simulink model "mmc_model"  (R2023b)
settings: Solver=VariableStepAuto  StartTime=0.0  StopTime=simulation.tsim  RelTol=1e-3
values from neighbouring files (symbols this model uses):
  ab0_to_cell = inv(cell_to_2ab0)    [init_mmc.m]
  cell_to_2ab0 = kron(abc_to_ab0, abc_to_ab0)    [init_mmc.m]
  grid_to_cell = kron(eye(3), ones(3, 1))    [init_mmc.m]
  J = [0 -1; 1 0]    [init_mmc.m]
  machine_to_cell = kron(ones(3, 1), eye(3))    [init_mmc.m]
  volt_to_cell = [      [          1 0 0 0 0 0 ... (first row only)    [init_mmc.m]
undefined symbols (not defined in the file or in its folder): avi, clc, cpu, ctrl, currentControl, DiscIntNeverNeededParam, gfl, grid, load2, loadStep, machine, mmc, pq_ctrl, simulation, soa, stiffGrid, sync, testScenario
libraries: library x17, spsThreePhaseSeriesRLCBranchLib x16, eeGeneralControl x15, spsControlledVoltageSourceLib x15, simulink x11, spsThreePhaseVIMeasurementLib x10, spsGroundLib x9, eeDiscretePi x8, simulink_extras x8, spsabctodq0Lib x8, spsThreePhaseBreakerLib x7, spsdq0toabcLib x5
(part 1 of 3)
settings Model: SimulationMode=accelerator  Creator=ma1155716  LastModifiedBy=ma1155716

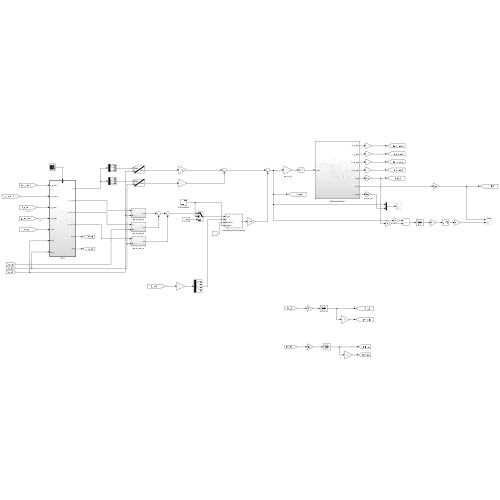
[thumbnail: Simulink's stored preview of the top-level diagram]
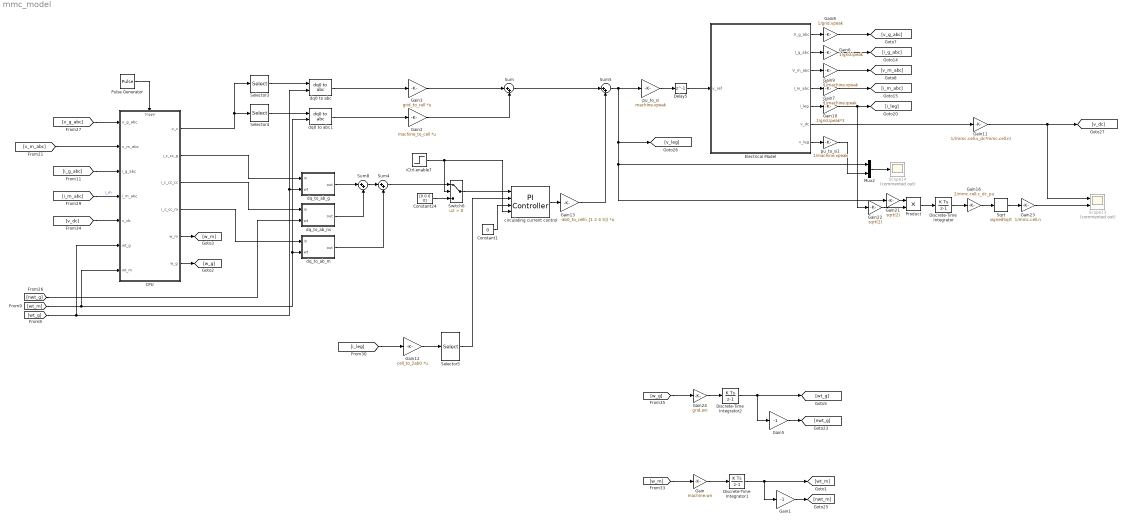
== system mmc_model ==
  CPU : Subsystem
  Constant1 : Constant  Value=0
  Constant24 : Constant  Value=[0 0 0 0]
  Delay5 : Delay  DelayLength=1  InitialCondition=0  SampleTime=simulation.ts
  Discrete-Time Integrator : DiscreteIntegrator  gainval=1  SampleTime=-1  ICPrevOutput=DiscIntNeverNeededParam  ICPrevScaledInput=DiscIntNeverNeededParam
  Discrete-Time Integrator1 : DiscreteIntegrator  gainval=1  SampleTime=-1  ICPrevOutput=DiscIntNeverNeededParam  ICPrevScaledInput=DiscIntNeverNeededParam
  Discrete-Time Integrator2 : DiscreteIntegrator  gainval=1  SampleTime=-1  ICPrevOutput=DiscIntNeverNeededParam  ICPrevScaledInput=DiscIntNeverNeededParam
  Electrical Model : Subsystem
  Gain : Gain  Gain=machine.wn
  Gain1 : Gain  Gain=-1
  Gain10 : Gain  Gain=1/grid.ipeak*3
  Gain11 : Gain  Gain=1/(mmc.cell.v_dc*mmc.cell.n)
  Gain12 : Gain  Gain=cell_to_2ab0  Multiplication=Matrix(K*u)
  Gain13 : Gain  Gain=-ab0_to_cell(:,[1 2 4 5])  Multiplication=Matrix(K*u)
  Gain16 : Gain  Gain=2/mmc.cell.c_dc_pu
  Gain2 : Gain  Gain=machine_to_cell  Multiplication=Matrix(K*u)
  Gain21 : Gain  Gain=sqrt(2)
  Gain22 : Gain  Gain=sqrt(2)
  Gain23 : Gain  Gain=1/mmc.cell.n
  Gain24 : Gain  Gain=grid.wn
  Gain3 : Gain  Gain=grid_to_cell  Multiplication=Matrix(K*u)
  Gain5 : Gain  Gain=-1
  Gain6 : Gain  Gain=1/grid.ipeak
  Gain7 : Gain  Gain=1/machine.ipeak
  Gain8 : Gain  Gain=1/grid.vpeak
  Gain9 : Gain  Gain=1/machine.vpeak
  Mux2 : Mux  Inputs=2
  Product : Product
  Pulse Generator : DiscretePulseGenerator  PulseType=Time based  Period=cpu.ts  PulseWidth=50
  Scope13 : Scope  Commented=on  NumInputPorts=2
  Scope14 : Scope  Commented=on
  Selector3 : Selector  InputPortWidth=5  IndexOptions=Index vector (dialog)  Indices=[1 2 5]  OutputSizes=1
  Selector4 : Selector  InputPortWidth=5  IndexOptions=Index vector (dialog)  Indices=[3 4 5]  OutputSizes=1
  Selector5 : Selector  InputPortWidth=9  IndexOptions=Index vector (dialog)  Indices=[1 2 4 5]  OutputSizes=1
  Sqrt : Sqrt  Operator=signedSqrt
  Sum{,4..5,8} (4 alike) : Sum  Inputs=|++
  Switch6 : Switch  Criteria=u2 > Threshold  SaturateOnIntegerOverflow=off  InputSameDT=off
  circulating current control : library/PI Controller  VariantControl=overcurr_ctrl.sel==1  kp=ctrl.grid.ictrl.kp  ti=1e6  Kaw=1
  dq0 to abc : spsdq0toabcLib/dq0 to abc  Alignment=Aligned with phase A axis
  dq0 to abc1 : spsdq0toabcLib/dq0 to abc  Alignment=Aligned with phase A axis
  dq_to_ab_g : Subsystem
  dq_to_ab_m : Subsystem
  dq_to_ab_ns : Subsystem
  iCtrl.enable7 : Step  Time=ctrl.grid.ictrl.enable
  pu_to_si : Gain  Gain=machine.vpeak
  pu_to_si1 : Gain  Gain=1/machine.vpeak
  wires:
  Electrical Model/2(I_g_abc) -> Gain6/1
  Electrical Model/4(I_m_abc) -> Gain7/1
  Pulse Generator/1 -> CPU/Trigger
  Discrete-Time Integrator2/1 -> [wt_g], Gain5/1
  Electrical Model/1(V_g_abc) -> Gain8/1
  Electrical Model/3(V_m_abc) -> Gain9/1
  dq0 to abc/1 -> Gain3/1
  dq0 to abc1/1 -> Gain2/1
  Selector3/1 -> dq0 to abc/1
  Selector4/1 -> dq0 to abc1/1
  CPU/1(v_c) -> Selector4/1, Selector3/1
  Gain3/1 -> Sum/1
  [i_g_abc] -> CPU/3(i_g_abc)
  pu_to_si/1 -> Delay5/1
  Electrical Model/5(i_leg) -> Gain10/1
  Gain6/1 -> [i_g_abc]
  Gain7/1 -> [i_m_abc]
  Gain8/1 -> [v_g_abc]
  Gain9/1 -> [v_m_abc]
  Gain10/1 -> Gain22/1, [i_leg]
  Gain5/1 -> [nwt_g]
  Discrete-Time Integrator1/1 -> [wt_m], Gain1/1
  Gain1/1 -> [nwt_m]
  Product/1 -> Discrete-Time Integrator/1
  [i_leg] -> Gain12/1
  Gain12/1 -> Selector5/1
  Discrete-Time Integrator/1 -> Gain16/1
  Gain16/1 -> Sqrt/1
  [v_dc] -> CPU/5(v_dc)
  Gain23/1 -> Scope13/2
  CPU/2(i_c_cc_g) -> dq_to_ab_g/1(in)
  [nwt_g] -> dq_to_ab_ns/2(wt)
  CPU/3(i_c_cc_cc) -> dq_to_ab_ns/1(in)
  CPU/4(i_c_cc_m) -> dq_to_ab_m/1(in)
  dq_to_ab_g/1(out) -> Sum8/1
  Sum8/1 -> Sum4/1
  dq_to_ab_ns/1(out) -> Sum8/2
  dq_to_ab_m/1(out) -> Sum4/2
  [wt_g] -> CPU/6(wt_g), dq0 to abc/2, dq_to_ab_g/2(wt)
  [wt_m] -> CPU/7(wt_m), dq_to_ab_m/2(wt), dq0 to abc1/2
  Constant1/1 -> circulating current control/3
  Sum4/1 -> Switch6/1
  Switch6/1 -> circulating current control/1
  iCtrl.enable7/1 -> Switch6/2, circulating current control/4
  Constant24/1 -> Switch6/3
  Sum/1 -> Sum5/1
  circulating current control/1 -> Gain13/1
  Gain11/1 -> [v_dc], Scope13/1
  Electrical Model/6(v_dc) -> Gain11/1
  Gain21/1 -> Product/1
  Gain22/1 -> Product/2
  Sqrt/1 -> Gain23/1
  Sum5/1 -> pu_to_si/1, [v_leg], Gain21/1, Mux2/1
  Electrical Model/7(v_leg) -> pu_to_si1/1
  pu_to_si1/1 -> Mux2/2
  Mux2/1 -> Scope14/1
  Gain2/1 -> Sum/2
  Selector5/1 -> circulating current control/2
  [i_m_abc] -> CPU/4(i_m_abc)  "i_m"
  CPU/5(w_m) -> [w_m]
  Gain/1 -> Discrete-Time Integrator1/1
  [w_m] -> Gain/1
  [v_g_abc] -> CPU/1(v_g_abc)
  Gain24/1 -> Discrete-Time Integrator2/1
  CPU/6(w_g) -> [w_g]
  [w_g] -> Gain24/1
  Gain13/1 -> Sum5/2
  Delay5/1 -> Electrical Model/1(v_ref)
  [v_m_abc] -> CPU/2(v_m_abc)

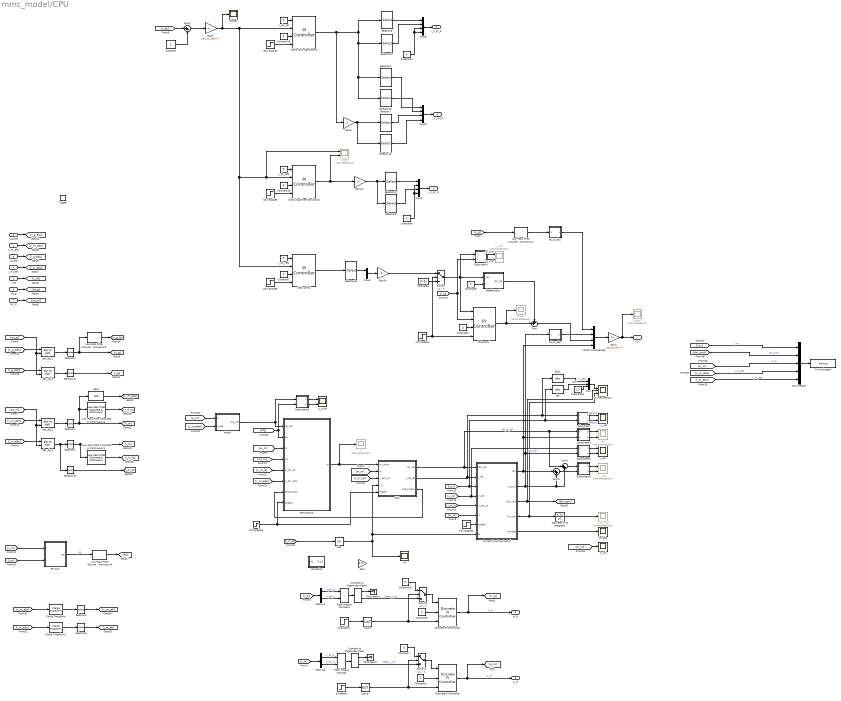
== system mmc_model/CPU ==
  v_g_abc : Inport
  v_m_abc : Inport  Port=2
  i_g_abc : Inport  Port=3
  i_m_abc : Inport  Port=4
  v_dc : Inport  Port=5
  wt_g : Inport  Port=6
  wt_m : Inport  Port=7
  Trigger : TriggerPort  VariantControl=(inherit)
  Abs : Abs  SaturateOnIntegerOverflow=off
  Bus Creator : BusCreator  Inputs=5
  Clarke Transform : eeTransforms/Clarke Transform  PowerInvariant=off
      settings: LibrarySourceBlock=|
      | ee_sl_lib/Mathematical
      | Transforms/Clarke Transform
  Clarke Transform1 : eeTransforms/Clarke Transform  PowerInvariant=off
      settings: LibrarySourceBlock=|
      | ee_sl_lib/Mathematical
      | Transforms/Clarke Transform
  Complex to Magnitude-Angle : ComplexToMagnitudeAngle
  Complex to Magnitude-Angle1 : ComplexToMagnitudeAngle
  Constant : Constant
  Constant{1..4,7..10,18..19} (10 alike) : Constant  Value=0
  Constant12 : Constant  Value=1.3
  Constant5 : Constant
  Constant6 : Constant  Value=[0 0]
  Current Limiting Control : Subsystem  Variant=on
  Demux1 : Demux  Outputs=2
  Demux6 : Demux  Outputs=2
  Discrete PI Controller : eeDiscretePi/Discrete PI Controller  Kp=ctrl.machine.pll.kp  Ki=ctrl.machine.pll.ti  Kaw=1  x0=ctrl.machine.pll.w0  Ts=-1
      settings: LibrarySourceBlock=ee_sl_lib/General Control/Discrete PI Controller
  Discrete PI Controller1 : eeDiscretePi/Discrete PI Controller  Kp=ctrl.grid.pll.kp  Ki=ctrl.grid.pll.ti  Kaw=1  x0=ctrl.grid.pll.w0  Ts=-1
      settings: LibrarySourceBlock=ee_sl_lib/General Control/Discrete PI Controller
  Discrete-Time Integrator : DiscreteIntegrator  gainval=1  SampleTime=-1  ICPrevOutput=DiscIntNeverNeededParam  ICPrevScaledInput=DiscIntNeverNeededParam
  GFM Control : Subsystem  Variant=on
  Gain : Gain  Gain=1.5
  Gain1 : Gain  Gain=volt_to_cell  Multiplication=Matrix(K*u)
  Gain12 : Gain  Gain=-1
  Gain14 : Gain  Gain=-1
  Gain5 : Gain  Gain=cell_to_2ab0  Multiplication=Matrix(K*u)
  Gain6 : Gain  Gain=-1
  Low-Pass Filter (Discrete or Continuous){1..4} (4 alike) : eeGeneralControl/Low-Pass Filter (Discrete or Continuous)  K=1  T=0.01  B=inf  A=-inf  init_option=Inherited from block input  x0=0  Ts=-1
  Low-Pass Filter (Discrete or Continuous)6 : eeGeneralControl/Low-Pass Filter (Discrete or Continuous)  K=1  T=0.1  B=inf  A=-inf  init_option=Inherited from block input  x0=0  Ts=-1
  Mux : Mux  Inputs=3
  Mux10 : Mux
  Mux6 : Mux  Inputs=2
  Mux8 : Mux
  Mux9 : Mux
  NOT1 : Logic  Operator=NOT  IconShape=distinctive  AllPortsSameDT=off  OutDataTypeStr=boolean
  NOT2 : Logic  Operator=NOT  IconShape=distinctive  AllPortsSameDT=off  OutDataTypeStr=boolean
  PQ Calc : Subsystem
  Real-Imag to Complex : RealImagToComplex
  Real-Imag to Complex1 : RealImagToComplex
  SOA : Subsystem
  Scope1 : Scope
  Scope5 : Scope  Commented=on
  Scope7 : Scope  Commented=on
  Scope8 : Scope  Commented=on  NumInputPorts=2
  Selector{1..5,17} (6 alike) : Selector  InputPortWidth=3  IndexOptions=Index vector (dialog)  Indices=[1 2]  OutputSizes=1
  Selector10 : Selector  InputPortWidth=9  IndexOptions=Index vector (dialog)  Indices=[8]  OutputSizes=1
  Selector11 : Selector  InputPortWidth=3  IndexOptions=Index vector (dialog)  Indices=[3]  OutputSizes=1
  Selector12 : Selector  InputPortWidth=9  IndexOptions=Index vector (dialog)  Indices=[3]  OutputSizes=1
  Selector13 : Selector  InputPortWidth=9  IndexOptions=Index vector (dialog)  Indices=[2]  OutputSizes=1
  Selector14 : Selector  InputPortWidth=9  IndexOptions=Index vector (dialog)  Indices=[5]  OutputSizes=1
  Selector15 : Selector  InputPortWidth=9  IndexOptions=Index vector (dialog)  Indices=[9]  OutputSizes=1
  Selector6 : Selector  InputPortWidth=9  IndexOptions=Index vector (dialog)  Indices=[1]  OutputSizes=1
  Selector7 : Selector  InputPortWidth=9  IndexOptions=Index vector (dialog)  Indices=[4]  OutputSizes=1
  Selector8 : Selector  InputPortWidth=9  IndexOptions=Index vector (dialog)  Indices=[7]  OutputSizes=1
  Selector9 : Selector  InputPortWidth=9  IndexOptions=Index vector (dialog)  Indices=[6]  OutputSizes=1
  Subsystem : Subsystem
  Subsystem1 : Subsystem
  Subsystem2 : Subsystem
  Subsystem3 : Subsystem
  Subsystem5 : Subsystem
  Subsystem6 : Subsystem
  Sum : Sum  Inputs=++|
  Sum1 : Sum  Inputs=|+-
  Sum3 : Sum  Inputs=|++
  Sum4 : Sum  Inputs=|++
  Switch : Switch  Criteria=u2 > Threshold  SaturateOnIntegerOverflow=off  InputSameDT=off
  Switch1 : Switch  Criteria=u2 > Threshold  SaturateOnIntegerOverflow=off  InputSameDT=off
  Switch2 : Switch  Criteria=u2 > Threshold  SaturateOnIntegerOverflow=off  InputSameDT=off
  Terminator1 : Terminator
  Terminator7 : Terminator
  To Workspace : ToWorkspace  VariableName=simout  SaveFormat=Timeseries  SampleTime=-1
  Vector Concatenate : Concatenate  NumInputs=4
  ab_to_ab0 : Subsystem
  ab_to_ab1 : Subsystem
  abc_dq_{1..4} (4 alike) : spsabctodq0Lib/abc to dq0  Alignment=Aligned with phase A axis
  abs : library/abs  SystemSampleTime=-1  VariantActivationTime=update diagram  AllowFlexibleInterface=on  Latency=0  AutoFrameSizeCalculation=off
  abs1 : library/abs  SystemSampleTime=-1  VariantActivationTime=update diagram  AllowFlexibleInterface=on  Latency=0  AutoFrameSizeCalculation=off
  abs3 : library/abs  SystemSampleTime=-1  VariantActivationTime=update diagram  AllowFlexibleInterface=on  Latency=0  AutoFrameSizeCalculation=off
  correction : Subsystem
  dm : Scope  Commented=on  NumInputPorts=2
  droop : Subsystem
  feedforward : Subsystem
  i0 : Scope
  iCtrl.enable : Step  Time=ctrl.grid.ictrl.enable
  iCtrl.enable1 : Step  Time=ctrl.machine.ictrl.enable
  iCtrl.enable2 : Step  Time=ctrl.machine.ictrl.enable
  iCtrl.enable3 : Step  Time=ctrl.grid.ictrl.enable
  iCtrl.enable4 : Step  Time=ctrl.grid.ictrl.enable
  iCtrl.enable5 : Step  Time=grid.breaker_close
  iG Control : library/PI Controller  VariantControl=overcurr_ctrl.sel==1  kp=ctrl.grid.ictrl.kp  ti=ctrl.grid.ictrl.ti  Kaw=1
  i_i_ref : Scope  NumInputPorts=2
  i_i_ref1 : Scope  Commented=on  NumInputPorts=2
  lambda : Scope
  m : Scope  Commented=on
  p_p-ref : Scope  NumInputPorts=2
  "pll.enable " : Step  Time=ctrl.grid.pll.enable
  pll.enable 1 : Step  Time=ctrl.grid.pll.enable
  sf interventions : Scope  NumInputPorts=3
  vCells Grid-side Control : library/PI Controller  VariantControl=overcurr_ctrl.sel==1  kp=ctrl.vdcctrl.kp  ti=ctrl.vdcctrl.ti  Kaw=1
  vCells Machine-side Control : library/PI Controller  VariantControl=overcurr_ctrl.sel==1  kp=ctrl.vdcctrl.kp  ti=ctrl.vdcctrl.ti*machine.fn/grid.fn  Kaw=1
  vDC control : library/PI Controller  VariantControl=overcurr_ctrl.sel==1  kp=ctrl.vdcctrl.kp  ti=ctrl.vdcctrl.ti  Kaw=1
  v_conv : Scope  Commented=on  NumInputPorts=2
  v_dc_ref : Constant  Value=0
  v_dc_ref1 : Constant  Value=0
  v_dc_ref2 : Constant  Value=0
  v_pcc : Scope  NumInputPorts=2
  v_pcc_diff : Scope  Commented=on
  w_m1 : Scope
  v_c : Outport
  i_c_cc_g : Outport  Port=2
  i_c_cc_cc : Outport  Port=3
  i_c_cc_m : Outport  Port=4
  w_m : Outport  Port=5
  w_g : Outport  Port=6
  wires:
  Switch/1 -> Subsystem1/1(x), feedforward/1(i_dq), iG Control/1
  Constant2/1 -> iG Control/3
  Vector Concatenate/1 -> Gain1/1
  Gain1/1 -> Scope5/1, v_c/1
  [i_g] -> iG Control/2, Subsystem1/2(y)
  Low-Pass Filter (Discrete or Continuous)2/1 -> ab_to_ab1/1(v_pcc_f)
  feedforward/1(dm_dq) -> Sum/1
  Constant5/1 -> feedforward/2(w)
  Constant6/1 -> Switch/3
  Sum/1 -> Vector Concatenate/3
  iG Control/1 -> Scope7/1, Sum/2
  iCtrl.enable/1 -> Switch/2, iG Control/4
  iCtrl.enable2/1 -> Current Limiting Control/7(enable)
  Mux8/1 -> i_c_cc_g/1
  v_dc_ref/1 -> vCells Grid-side Control/1
  iCtrl.enable4/1 -> vCells Grid-side Control/4
  Constant18/1 -> vCells Grid-side Control/3
  Selector6/1 -> Mux10/1
  Selector7/1 -> Mux10/3
  Selector8/1 -> Mux8/1
  Mux10/1 -> i_c_cc_cc/1
  Selector10/1 -> Mux8/2
  Mux9/1 -> i_c_cc_m/1
  vCells Grid-side Control/1 -> Gain6/1, Selector13/1, Selector6/1, Selector10/1, Selector8/1
  Selector13/1 -> Mux10/2
  Selector14/1 -> Mux10/4
  Selector12/1 -> Mux9/1
  Selector9/1 -> Mux9/3
  Selector15/1 -> Mux6/1
  Gain14/1 -> Switch/1
  v_dc_ref1/1 -> vCells Machine-side Control/1
  Constant19/1 -> vCells Machine-side Control/3
  iCtrl.enable3/1 -> vCells Machine-side Control/4
  Sum1/1 -> Gain5/1
  vCells Machine-side Control/1 -> Scope8/2, Gain12/1
  Mux6/1 -> Gain14/1
  v_dc_ref2/1 -> vDC control/1
  Constant1/1 -> vDC control/3
  iCtrl.enable5/1 -> vDC control/4
  vDC control/1 -> Selector15/1
  SOA/1(dm_dq) -> Sum4/1, Subsystem5/1(x), Current Limiting Control/1(dm_ref)  "dv_m_ref"
  Current Limiting Control/5(lambda) -> lambda/1
  Current Limiting Control/3(dm_corr) -> [dm_corr], sf interventions/2  "dm_corr"
  [v_m_lp] -> Current Limiting Control/5(v_pcc_lp)
  Constant/1 -> Sum1/2
  Current Limiting Control/2(v_pcc_f) -> ab_to_ab0/1(v_pcc_f), Subsystem2/2(y), Sum4/2, Sum3/2
  ab_to_ab0/1(Out1) -> Vector Concatenate/2
  Subsystem/1(d) -> i_i_ref/1  "irefd_id"
  Subsystem/2(q) -> i_i_ref/2  "irefq_iq"
  Subsystem1/2(q) -> i_i_ref1/2  "iq_iqref"
  Subsystem1/1(d) -> i_i_ref1/1  "id_idref"
  Constant4/1 -> Mux8/3, Mux8/4
  Constant8/1 -> Mux9/2, Mux9/4
  Gain5/1 -> vCells Grid-side Control/2, Scope8/1, vCells Machine-side Control/2, vDC control/2, Scope1/1
  Gain12/1 -> Selector9/1, Selector12/1
  Gain6/1 -> Selector7/1, Selector14/1
  "pll.enable "/1 -> NOT1/1
  Switch1/1 -> Discrete PI Controller/1
  Real-Imag to Complex/1 -> Complex to Magnitude-Angle/1
  Complex to Magnitude-Angle/1 -> Terminator7/1
  Constant3/1 -> Discrete PI Controller/2
  Demux6/1 -> Real-Imag to Complex/1  "v_pll_d"
  Constant7/1 -> Switch1/1
  Discrete PI Controller/1 -> [w_m], w_m/1  "w_m"
  Constant10/1 -> Switch2/1
  NOT2/1 -> Discrete PI Controller1/3, Switch2/2
  Demux1/1 -> Real-Imag to Complex1/1  "v_pll_d"
  Real-Imag to Complex1/1 -> Complex to Magnitude-Angle1/1
  Complex to Magnitude-Angle1/1 -> Terminator1/1
  Complex to Magnitude-Angle1/2 -> Switch2/3  "theta_v_pll"
  Switch2/1 -> Discrete PI Controller1/1
  Demux1/2 -> Real-Imag to Complex1/2  "v_pll_q"
  Discrete PI Controller1/1 -> w_g/1, [w_g]  "w_g"
  pll.enable 1/1 -> NOT2/1
  Constant9/1 -> Discrete PI Controller1/2
  [v_m] -> Demux6/1
  Selector3/1 -> [v_g], Low-Pass Filter (Discrete or Continuous)3/1
  [v_g] -> Demux1/1
  NOT1/1 -> Switch1/2, Discrete PI Controller/3
  Current Limiting Control/1(dm) -> Vector Concatenate/4, Subsystem5/2(y), Sum3/1
  Subsystem2/1(d) -> v_pcc/1
  Subsystem2/2(q) -> v_pcc/2
  Subsystem5/1(d) -> dm/1
  Subsystem5/2(q) -> dm/2
  Mux/1 -> sf interventions/1
  Constant12/1 -> Mux/3
  abs1/1 -> Mux/1  "ir_abs"
  abs/1 -> Mux/2  "i_abs"
  Demux6/2 -> Real-Imag to Complex/2  "v_pll_q"
  Sum3/1 -> Subsystem6/2(y)
  Sum4/1 -> Subsystem6/1(x)
  Subsystem6/1(d) -> v_conv/1
  Subsystem6/2(q) -> v_conv/2
  Complex to Magnitude-Angle/2 -> Switch1/3  "theta_v_pll"
  [w_m] -> w_m1/1
  Current Limiting Control/4(dv_corr) -> sf interventions/3, Discrete-Time Integrator/1
  Discrete-Time Integrator/1 -> v_pcc_diff/1
  [w_m] -> Current Limiting Control/6(w)
  [w_m] -> SOA/2(w)
  [v_g] -> Low-Pass Filter (Discrete or Continuous)2/1
  wt_m/1 -> [wt_m]
  wt_g/1 -> [wt_g]
  abc_dq_1/1 -> Selector3/1
  [wt_g] -> abc_dq_1/2, abc_dq_3/2
  abc_dq_3/1 -> Selector17/1
  [wt_m] -> abc_dq_2/2, abc_dq_4/2
  abc_dq_2/1 -> Selector1/1
  abc_dq_4/1 -> Selector11/1, Selector2/1
  [v_dc] -> Sum1/1
  v_dc/1 -> [v_dc]
  [i_m_abc] -> abc_dq_4/1
  i_m_abc/1 -> [i_m_abc]
  [i_g_abc] -> abc_dq_3/1
  i_g_abc/1 -> [i_g_abc]
  [v_m_abc] -> abc_dq_2/1
  v_m_abc/1 -> [v_m_abc]
  [v_g_abc] -> abc_dq_1/1
  v_g_abc/1 -> [v_g_abc]
  Selector17/1 -> [i_g]
  Low-Pass Filter (Discrete or Continuous)3/1 -> [v_g_lp]
  Low-Pass Filter (Discrete or Continuous)4/1 -> [v_m_lp]
  abs3/1 -> [v_m_abs]
  ab_to_ab1/1(Out1) -> Vector Concatenate/1
  GFM Control/1(m) -> m/1, SOA/1(m_unlim)
  [v_m_lp] -> GFM Control/5(v_pcc_lp)
  [v_m_lp] -> SOA/3(v_pcc_lp)
  [v_m_abs] -> GFM Control/6(v_pcc_abs)
  droop/1(PQ_ref) -> Subsystem3/1(x), GFM Control/1(pq_ref)
  SOA/3(antiwindup) -> GFM Control/7(antiwindup)
  [PQ] -> Subsystem3/2(y), GFM Control/2(pq)
  iCtrl.enable1/1 -> SOA/5(enable), GFM Control/8(enable)
  PQ Calc/1(PQ) -> Low-Pass Filter (Discrete or Continuous)6/1  "PQ"
  [v_m] -> PQ Calc/1(v)
  [i_m] -> PQ Calc/2(i)
  Low-Pass Filter (Discrete or Continuous)6/1 -> [PQ]
  [w_m] -> droop/1(w)
  [v_m_abs] -> droop/2(u_abs)
  Subsystem3/2(q) -> p_p-ref/2
  Subsystem3/1(d) -> p_p-ref/1
  [w_m] -> GFM Control/3(w)
  [wt_m] -> GFM Control/4(wt)
  [v_m_abc] -> Clarke Transform/1
  Clarke Transform/1 -> Selector4/1
  Selector4/1 -> [v_m_ab]
  [i_m_abc] -> Clarke Transform1/1
  Clarke Transform1/1 -> Selector5/1
  Selector5/1 -> [i_m_ab]
  Low-Pass Filter (Discrete or Continuous)1/1 -> [i_m_lp]
  Selector1/1 -> [v_m], abs3/1, Low-Pass Filter (Discrete or Continuous)4/1
  Selector11/1 -> [i_m_0]
  Selector2/1 -> [i_m], Low-Pass Filter (Discrete or Continuous)1/1
  [i_m] -> Current Limiting Control/3(i), abs/1, Subsystem/2(y)
  SOA/2(i_ref_dq) -> Subsystem/1(x), abs1/1, Current Limiting Control/2(i_ref)
  Abs/1 -> SOA/4(i_0), Current Limiting Control/8(i0), i0/1
  [i_m_abc] -> Bus Creator/5  "i_m_abc"
  [w_m] -> Bus Creator/3  "w_m"
  Bus Creator/1 -> To Workspace/1
  [dm_corr] -> Bus Creator/2  "dm_corr"
  [v_m_abc] -> Bus Creator/4  "v_m_abc"
  [i_m] -> Bus Creator/1  "i_m"
  [v_m] -> Subsystem2/1(x), Current Limiting Control/4(v_pcc)
  [i_m_0] -> Abs/1

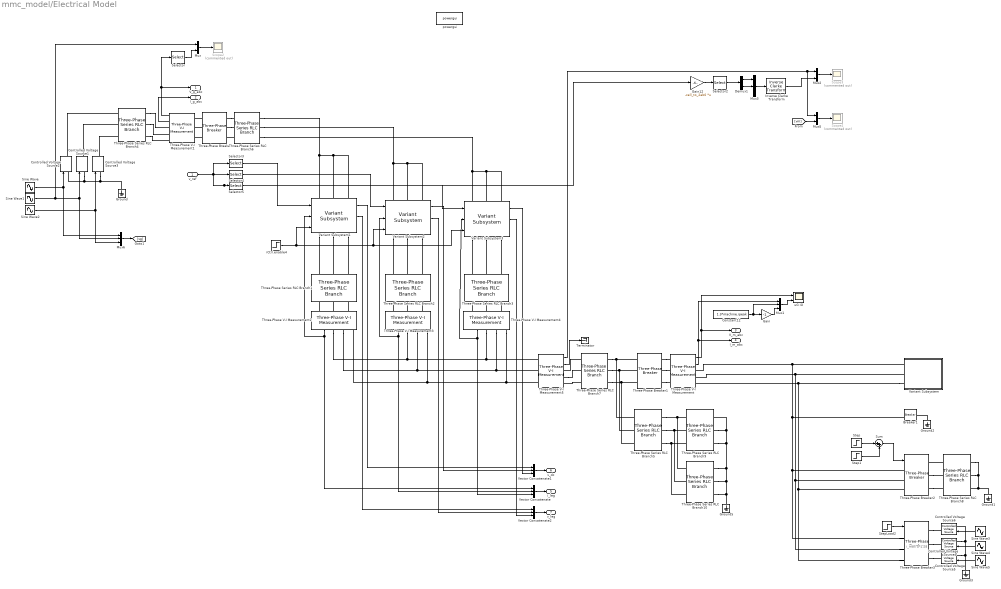
== system mmc_model/Electrical Model ==
  note: i_max = 1.28
  v_ref : Inport
  Breaker1 : spsBreakerLib/Breaker  InitialState=0  SwitchingTimes="[1/60  5/60]"  External=on  BreakerResistance=0.01  SnubberResistance=1e6  SnubberCapacitance=inf  Measurements=None  MoreParameters=on  NoBreakLoop=off
  Constant12 : Constant  Value=1.3*machine.ipeak
  Controlled Voltage Source{1..6} (6 alike) : spsControlledVoltageSourceLib/Controlled Voltage Source  Initialize=on  Source_Type=AC  Amplitude=0  Phase=0  Frequency=0  Measurements=None
  Demux1 : Demux  Outputs=2
  Gain : Gain  Gain=-1
  Gain12 : Gain  Gain=-cell_to_2ab0  Multiplication=Matrix(K*u)
  Ground{,1..3,5} (5 alike) : spsGroundLib/Ground  LConnTagsString=a
  Inverse Clarke Transform : eeTransforms/Inverse Clarke Transform  PowerInvariant=off
      settings: LibrarySourceBlock=|
      | ee_sl_lib/Mathematical
      | Transforms/Inverse
      | Clarke Transform
  Mux : Mux  Inputs=2
  Mux1 : Mux  Inputs=[3 1 1]
  Mux2 : Mux  Inputs=2
  Mux3 : Mux  Inputs=3
  Mux5 : Mux  Inputs=2
  Mux6 : Mux  Inputs=3
  Scope2 : Scope  Commented=on
  Scope3 : Scope  Commented=on
  Scope4 : Scope  Commented=on
  Selector : Selector  InputPortWidth=3  IndexOptions=Index vector (dialog)  Indices=[2]  OutputSizes=1
  Selector2 : Selector  InputPortWidth=9  IndexOptions=Index vector (dialog)  Indices=[7 8]  OutputSizes=1
  Selector3 : Selector  InputPortWidth=9  IndexOptions=Index vector (dialog)  Indices=[1 2 3]  OutputSizes=1
  Selector4 : Selector  InputPortWidth=9  IndexOptions=Index vector (dialog)  Indices=[4 5 6]  OutputSizes=1
  Selector5 : Selector  InputPortWidth=9  IndexOptions=Index vector (dialog)  Indices=[7 8 9]  OutputSizes=1
  Sine Wave : Sin  Amplitude=grid.vpeak  Frequency=grid.wn  Phase=pi/2  SampleTime=0
  Sine Wave1 : Sin  Amplitude=grid.vpeak  Frequency=grid.wn  Phase=pi/2-2*pi/3  SampleTime=0
  Sine Wave2 : Sin  Amplitude=grid.vpeak  Frequency=grid.wn  Phase=pi/2+2*pi/3  SampleTime=0
  Sine Wave3 : Sin  Amplitude=stiffGrid.vpeak  Frequency=stiffGrid.w  Phase=pi/2  SampleTime=0
  Sine Wave4 : Sin  Amplitude=stiffGrid.vpeak  Frequency=stiffGrid.w  Phase=pi/2-2*pi/3  SampleTime=0
  Sine Wave5 : Sin  Amplitude=stiffGrid.vpeak  Frequency=stiffGrid.w  Phase=pi/2+2*pi/3  SampleTime=0
  Step : Step  Time=loadStep.stepDown  SampleTime=0
  Step1 : Step  Time=loadStep.stepUp  After=-1  SampleTime=0
  StepLoad2 : Step  Time=sync.breaker_open  Before=1  After=0  SampleTime=0
  Sum : Sum  Inputs=|++
  Terminator : Terminator
  Three-Phase Series RLC Branch1 : spsThreePhaseSeriesRLCBranchLib/Three-Phase Series RLC Branch  LConnTagsString=A|B|C  RConnTagsString=A|B|C  BranchType=RL  Resistance=mmc.r_leg_si  Inductance=mmc.l_leg_si  Capacitance=1e-6  Measurements=None
  Three-Phase Series RLC Branch10 : spsThreePhaseSeriesRLCBranchLib/Three-Phase Series RLC Branch  LConnTagsString=A|B|C  RConnTagsString=A|B|C  BranchType=L  Resistance=machine.filter.r_si  Inductance=machine.filter.l_si  Capacitance=machine.filter.c_si  Measurements=None
  Three-Phase Series RLC Branch2 : spsThreePhaseSeriesRLCBranchLib/Three-Phase Series RLC Branch  LConnTagsString=A|B|C  RConnTagsString=A|B|C  BranchType=RL  Resistance=mmc.r_leg_si  Inductance=mmc.l_leg_si  Capacitance=1e-6  Measurements=None
  Three-Phase Series RLC Branch3 : spsThreePhaseSeriesRLCBranchLib/Three-Phase Series RLC Branch  LConnTagsString=A|B|C  RConnTagsString=A|B|C  BranchType=RL  Resistance=mmc.r_leg_si  Inductance=mmc.l_leg_si  Capacitance=1e-6  Measurements=None
  Three-Phase Series RLC Branch4 : spsThreePhaseSeriesRLCBranchLib/Three-Phase Series RLC Branch  LConnTagsString=A|B|C  RConnTagsString=A|B|C  BranchType=RL  Resistance=grid.tr.r_si*0.1  Inductance=grid.tr.l_si*0.1  Capacitance=1e-6  Measurements=None
  Three-Phase Series RLC Branch5 : spsThreePhaseSeriesRLCBranchLib/Three-Phase Series RLC Branch  LConnTagsString=A|B|C  RConnTagsString=A|B|C  BranchType=C  Resistance=machine.filter.r_si  Inductance=loadStep.l_si  Capacitance=machine.filter.c_si  Measurements=None
  Three-Phase Series RLC Branch6 : spsThreePhaseSeriesRLCBranchLib/Three-Phase Series RLC Branch  LConnTagsString=A|B|C  RConnTagsString=A|B|C  BranchType=RL  Resistance=grid.tr.r_si  Inductance=grid.tr.l_si  Capacitance=1e-6  Measurements=None
  Three-Phase Series RLC Branch7 : spsThreePhaseSeriesRLCBranchLib/Three-Phase Series RLC Branch  LConnTagsString=A|B|C  RConnTagsString=A|B|C  BranchType=RL  Resistance=machine.tr.r_si  Inductance=machine.tr.l_si  Capacitance=1e-6  Measurements=None
  Three-Phase Series RLC Branch8 : spsThreePhaseSeriesRLCBranchLib/Three-Phase Series RLC Branch  LConnTagsString=A|B|C  RConnTagsString=A|B|C  BranchType=RL  Resistance=loadStep.r_si  Inductance=loadStep.l_si  Capacitance=1e-6  Measurements=None
  Three-Phase Series RLC Branch9 : spsThreePhaseSeriesRLCBranchLib/Three-Phase Series RLC Branch  LConnTagsString=A|B|C  RConnTagsString=A|B|C  BranchType=R  Resistance=machine.filter.r_si  Inductance=loadStep.l_si  Capacitance=machine.filter.c_si  Measurements=None
  Three-Phase V-I Measurement{,1..5} (6 alike) : spsThreePhaseVIMeasurementLib/Three-Phase V-I Measurement  VoltageMeasurement=phase-to-ground  SetLabelV=off  LabelV=Vabc  Vpu=off  VpuLL=off  CurrentMeasurement=yes  SetLabelI=off  LabelI=Iabc  Ipu=off  Pbase=100e6  Vbase=500e3  OutputType=Complex  PhasorSimulation=off  PSBequivalent=0
  Three-Phase Breaker : spsThreePhaseBreakerLib/Three-Phase Breaker  InitialState=open  SwitchA=on  SwitchB=on  SwitchC=on  SwitchTimes=[grid.breaker_close]  External=off  BreakerResistance=0.01  SnubberResistance=1e6  SnubberCapacitance=inf  Measurements=None
  Three-Phase Breaker1 : spsThreePhaseBreakerLib/Three-Phase Breaker  InitialState=open  SwitchA=on  SwitchB=on  SwitchC=on  SwitchTimes=[machine.breaker_close]  External=off  BreakerResistance=0.01  SnubberResistance=1e6  SnubberCapacitance=inf  Measurements=None
  Three-Phase Breaker2 : spsThreePhaseBreakerLib/Three-Phase Breaker  InitialState=open  SwitchA=on  SwitchB=on  SwitchC=on  SwitchTimes=[machine.breaker_close]  External=on  BreakerResistance=0.01  SnubberResistance=1e6  SnubberCapacitance=inf  Measurements=None
  Three-Phase Breaker3 : spsThreePhaseBreakerLib/Three-Phase Breaker  InitialState=open  SwitchA=on  SwitchB=on  SwitchC=on  SwitchTimes=[machine.breaker_close]  External=on  BreakerResistance=0.01  SnubberResistance=1e6  SnubberCapacitance=inf  Measurements=None
  Variant Subsystem : Subsystem  Variant=on
  Variant Subsystem1 : library/Variant Subsystem  SystemSampleTime=-1  VariantActivationTime=update diagram  AllowFlexibleInterface=on  Latency=0  AutoFrameSizeCalculation=off
      settings: PortSchema="{\"entries\":[{\"content\":{\"sides\":[{\"content\":{\"connectorIds\":[\"In1\",\"In2\",\"In3\"]},\"type\":\"ConnectorPlacement.EquallySpacedRectSide\",\"uuid\":\"07cc1b48-4eec-48c8-b7e1-ba85327af049\"},{\"content\":{\"connectorIds\":[\"Out1\",\"Out2\",\"Out3\"],\"side\":\"RIGHT\"},\"type\":\"ConnectorPlacement.EquallySpacedRectSide\",\"uuid\":\"e630ccd2-bced-4562-b965-5ba67d1cb520\"},{\"content\":{\"connectorIds\":[\"LConn1\",\"LConn2\",\"LConn3\"],\"side\":\"TOP\"},\"type\":\"ConnectorPlacement.EquallySpacedRectSide\",\"uuid\":\"f7ee33a5-0b9e-482c-ae72-b6ca50f6d328\"},{\"content\":{\"connectorIds\":[\"RConn1\",\"RConn2\",\"RConn3\"],\"side\":\"BOTTOM\"},\"type\":\"ConnectorPlacement.EquallySpacedRectSide\",\"uuid\":\"76c11136-f7c0-446b-9aed-353e2cf8a045\"}]},\"type\":\"ConnectorPlacement.EquallySpacedConnector\",\"uuid\":\"ad2af07b-650a-4f66-848d-c3c749fafa1e\"}],\"packageUris\":[\"http://schema.mathworks.com/mf0/Connector/R2020b\"],\"version\":\"1.0\"}"
  Variant Subsystem2 : library/Variant Subsystem  SystemSampleTime=-1  VariantActivationTime=update diagram  AllowFlexibleInterface=on  Latency=0  AutoFrameSizeCalculation=off
      settings: PortSchema="{\"entries\":[{\"content\":{\"sides\":[{\"content\":{\"connectorIds\":[\"In1\",\"In2\",\"In3\"]},\"type\":\"ConnectorPlacement.EquallySpacedRectSide\",\"uuid\":\"07cc1b48-4eec-48c8-b7e1-ba85327af049\"},{\"content\":{\"connectorIds\":[\"Out1\",\"Out2\",\"Out3\"],\"side\":\"RIGHT\"},\"type\":\"ConnectorPlacement.EquallySpacedRectSide\",\"uuid\":\"e630ccd2-bced-4562-b965-5ba67d1cb520\"},{\"content\":{\"connectorIds\":[\"LConn1\",\"LConn2\",\"LConn3\"],\"side\":\"TOP\"},\"type\":\"ConnectorPlacement.EquallySpacedRectSide\",\"uuid\":\"f7ee33a5-0b9e-482c-ae72-b6ca50f6d328\"},{\"content\":{\"connectorIds\":[\"RConn1\",\"RConn2\",\"RConn3\"],\"side\":\"BOTTOM\"},\"type\":\"ConnectorPlacement.EquallySpacedRectSide\",\"uuid\":\"76c11136-f7c0-446b-9aed-353e2cf8a045\"}]},\"type\":\"ConnectorPlacement.EquallySpacedConnector\",\"uuid\":\"ad2af07b-650a-4f66-848d-c3c749fafa1e\"}],\"packageUris\":[\"http://schema.mathworks.com/mf0/Connector/R2020b\"],\"version\":\"1.0\"}"
  Variant Subsystem3 : library/Variant Subsystem  SystemSampleTime=-1  VariantActivationTime=update diagram  AllowFlexibleInterface=on  Latency=0  AutoFrameSizeCalculation=off
      settings: PortSchema="{\"entries\":[{\"content\":{\"sides\":[{\"content\":{\"connectorIds\":[\"In1\",\"In2\",\"In3\"]},\"type\":\"ConnectorPlacement.EquallySpacedRectSide\",\"uuid\":\"07cc1b48-4eec-48c8-b7e1-ba85327af049\"},{\"content\":{\"connectorIds\":[\"Out1\",\"Out2\",\"Out3\"],\"side\":\"RIGHT\"},\"type\":\"ConnectorPlacement.EquallySpacedRectSide\",\"uuid\":\"e630ccd2-bced-4562-b965-5ba67d1cb520\"},{\"content\":{\"connectorIds\":[\"LConn1\",\"LConn2\",\"LConn3\"],\"side\":\"TOP\"},\"type\":\"ConnectorPlacement.EquallySpacedRectSide\",\"uuid\":\"f7ee33a5-0b9e-482c-ae72-b6ca50f6d328\"},{\"content\":{\"connectorIds\":[\"RConn1\",\"RConn2\",\"RConn3\"],\"side\":\"BOTTOM\"},\"type\":\"ConnectorPlacement.EquallySpacedRectSide\",\"uuid\":\"76c11136-f7c0-446b-9aed-353e2cf8a045\"}]},\"type\":\"ConnectorPlacement.EquallySpacedConnector\",\"uuid\":\"ad2af07b-650a-4f66-848d-c3c749fafa1e\"}],\"packageUris\":[\"http://schema.mathworks.com/mf0/Connector/R2020b\"],\"version\":\"1.0\"}"
  Vector Concatenate : Concatenate  NumInputs=3
  Vector Concatenate1 : Concatenate  NumInputs=3
  Vector Concatenate2 : Concatenate  NumInputs=3
  iCtrl.enable4 : Step  Time=ctrl.grid.ictrl.enable
  powergui : spspowerguiLib/powergui  Priority=1  SimulationMode=Discrete  SampleTime=simulation.ts  frequency=60  Iterations=50  frequencyindice=0  Pbase=100e6  ErrMax=1e-4  UnitsV=kV  UnitsW=MW  buscounter=0  FunctionMessages=off  echomessages=off  EnableUseOfTLC=off  CurrentSourceSwitches=off  DisableSnubberDevices=off  DisableRonSwitches=off  DisableVfSwitches=off  DisplayEquations=off  AutomaticDiscreteSolvers=off  SolverType=Tustin/Backward Euler (TBE)  Interpol=off  ExternalGateDelay=off  methode=off  Ts=100  x0status=blocks  SPID=on  SwTol=0  HookPort=off  NonlinearTolerance=1e-4  nMaxIteration=100  ContinueOnMaxIteration=off  RestoreLinks=warning  ResistiveCurrentMeasurement=off  Frange=[0:2:500]  Ylog=off  Xlog=on  ShowGrid=off  save=off  variable=ZData  structure=0  ZoomFFT=off  StartTime=0.0  cycles=1  DisplayStyle=1  fundamental=60  FreqAxis=off  MaxFrequency=1000  frequencyindicesteady=1  RmsSteady=1  display=off
  uG iG : Scope  NumInputPorts=2
  V_g_abc : Outport
  I_g_abc : Outport  Port=2
  V_m_abc : Outport  Port=3
  I_m_abc : Outport  Port=4
  i_leg : Outport  Port=5
  v_dc : Outport  Port=6
  v_leg : Outport  Port=7
  wires:
  Sine Wave1/1 -> Mux/1, Controlled Voltage Source1/1, Mux6/2
  Sine Wave/1 -> Controlled Voltage Source2/1, Mux6/1
  Sine Wave2/1 -> Mux6/3, Controlled Voltage Source3/1
  Selector/1 -> Mux/2
  Mux/1 -> Scope2/1
  Three-Phase V-I Measurement2/2 -> Variant Subsystem1/2, Vector Concatenate/1
  Three-Phase V-I Measurement3/2 -> Variant Subsystem2/2, Vector Concatenate/2
  Three-Phase V-I Measurement4/2 -> Variant Subsystem3/2, Vector Concatenate/3
  Three-Phase V-I Measurement/1 -> V_m_abc/1, uG iG/1
  Three-Phase V-I Measurement/2 -> I_m_abc/1, Mux1/1
  Three-Phase V-I Measurement1/1 -> V_g_abc/1, Selector/1
  Three-Phase V-I Measurement1/2 -> I_g_abc/1
  Vector Concatenate/1 -> i_leg/1
  Variant Subsystem1/1 -> Vector Concatenate1/1
  Variant Subsystem2/1 -> Vector Concatenate1/2
  Variant Subsystem3/1 -> Vector Concatenate1/3
  Vector Concatenate1/1 -> v_dc/1
  Vector Concatenate2/1 -> v_leg/1
  Variant Subsystem1/2 -> Vector Concatenate2/1
  Variant Subsystem2/2 -> Vector Concatenate2/2
  Variant Subsystem3/2 -> Vector Concatenate2/3
  Three-Phase V-I Measurement5/1 -> Mux5/1, Mux2/1
  Mux2/1 -> Scope3/1
  v_ref/1 -> Gain12/1, Selector5/1, Selector4/1, Selector3/1
  Gain12/1 -> Selector2/1
  Selector2/1 -> Demux1/1
  Demux1/1 -> Mux3/1
  Demux1/2 -> Mux3/2
  Mux3/1 -> Inverse Clarke Transform/1
  Inverse Clarke Transform/1 -> Mux2/2
  iCtrl.enable4/1 -> Variant Subsystem1/3, Variant Subsystem3/3, Variant Subsystem2/3
  Selector3/1 -> Variant Subsystem1/1
  Selector4/1 -> Variant Subsystem2/1
  Selector5/1 -> Variant Subsystem3/1
  [vm] -> Mux5/2
  Mux5/1 -> Scope4/1
  Mux6/1 -> [vg]
  Sine Wave3/1 -> Controlled Voltage Source6/1
  Sine Wave4/1 -> Controlled Voltage Source4/1
  Sine Wave5/1 -> Controlled Voltage Source5/1
  StepLoad2/1 -> Three-Phase Breaker3/1
  Step/1 -> Sum/1
  Step1/1 -> Sum/2
  Three-Phase V-I Measurement5/2 -> Terminator/1
  Mux1/1 -> uG iG/2
  Constant12/1 -> Gain/1, Mux1/2
  Gain/1 -> Mux1/3
  Sum/1 -> Three-Phase Breaker2/1
  connections:
  Three-Phase Series RLC Branch6/RConn1 -- Variant Subsystem1/LConn1 -- Variant Subsystem1/LConn2 -- Variant Subsystem1/LConn3
  Ground/LConn1 -- Controlled Voltage Source2/LConn1 -- Controlled Voltage Source1/LConn1 -- Controlled Voltage Source3/LConn1
  Three-Phase Series RLC Branch6/RConn2 -- Variant Subsystem2/LConn1 -- Variant Subsystem2/LConn3 -- Variant Subsystem2/LConn2
  Three-Phase V-I Measurement2/RConn1 -- Three-Phase V-I Measurement3/RConn1 -- Three-Phase V-I Measurement5/LConn1 -- Three-Phase V-I Measurement4/RConn1
  Controlled Voltage Source1/RConn1 -- Three-Phase Series RLC Branch4/LConn2
  Three-Phase Series RLC Branch4/RConn1 -- Three-Phase V-I Measurement1/RConn1
  Breaker1/LConn1 -- Three-Phase Breaker3/LConn1 -- Three-Phase Breaker2/LConn1 -- Three-Phase V-I Measurement/RConn1 -- Variant Subsystem/LConn1
  Three-Phase Series RLC Branch6/RConn3 -- Variant Subsystem3/LConn1 -- Variant Subsystem3/LConn2 -- Variant Subsystem3/LConn3
  Three-Phase Series RLC Branch4/RConn3 -- Three-Phase V-I Measurement1/RConn3
  Variant Subsystem/LConn3 -- Three-Phase Breaker3/LConn3 -- Three-Phase Breaker2/LConn3 -- Three-Phase V-I Measurement/RConn3
  Three-Phase V-I Measurement2/RConn2 -- Three-Phase V-I Measurement3/RConn2 -- Three-Phase V-I Measurement5/LConn2 -- Three-Phase V-I Measurement4/RConn2
  Controlled Voltage Source3/RConn1 -- Three-Phase Series RLC Branch4/LConn3
  Three-Phase Series RLC Branch4/RConn2 -- Three-Phase V-I Measurement1/RConn2
  Controlled Voltage Source2/RConn1 -- Three-Phase Series RLC Branch4/LConn1
  Three-Phase V-I Measurement2/RConn3 -- Three-Phase V-I Measurement5/LConn3 -- Three-Phase V-I Measurement4/RConn3 -- Three-Phase V-I Measurement3/RConn3
  Three-Phase Breaker3/LConn2 -- Three-Phase Breaker2/LConn2 -- Three-Phase V-I Measurement/RConn2 -- Variant Subsystem/LConn2
  Three-Phase V-I Measurement2/LConn1 -- Three-Phase Series RLC Branch1/RConn1
  Three-Phase V-I Measurement2/LConn2 -- Three-Phase Series RLC Branch1/RConn2
  Three-Phase V-I Measurement2/LConn3 -- Three-Phase Series RLC Branch1/RConn3
  Three-Phase V-I Measurement3/LConn1 -- Three-Phase Series RLC Branch2/RConn1
  Three-Phase V-I Measurement3/LConn2 -- Three-Phase Series RLC Branch2/RConn2
  Three-Phase V-I Measurement3/LConn3 -- Three-Phase Series RLC Branch2/RConn3
  Three-Phase V-I Measurement4/LConn1 -- Three-Phase Series RLC Branch3/RConn1
  Three-Phase V-I Measurement4/LConn2 -- Three-Phase Series RLC Branch3/RConn2
  Three-Phase V-I Measurement4/LConn3 -- Three-Phase Series RLC Branch3/RConn3
  Three-Phase Breaker/RConn1 -- Three-Phase Series RLC Branch6/LConn1
  Three-Phase Breaker/RConn2 -- Three-Phase Series RLC Branch6/LConn2
  Three-Phase Series RLC Branch6/LConn3 -- Three-Phase Breaker/RConn3
  Three-Phase Breaker/LConn1 -- Three-Phase V-I Measurement1/LConn1
  Three-Phase Breaker/LConn2 -- Three-Phase V-I Measurement1/LConn2
  Three-Phase Breaker/LConn3 -- Three-Phase V-I Measurement1/LConn3
  Three-Phase Series RLC Branch7/RConn1 -- Three-Phase Series RLC Branch5/LConn1 -- Three-Phase Breaker1/LConn1
  Three-Phase Series RLC Branch7/RConn2 -- Three-Phase Series RLC Branch5/LConn2 -- Three-Phase Breaker1/LConn2
  Three-Phase Series RLC Branch7/RConn3 -- Three-Phase Series RLC Branch5/LConn3 -- Three-Phase Breaker1/LConn3
  Three-Phase Breaker1/RConn3 -- Three-Phase V-I Measurement/LConn3
  Three-Phase Breaker1/RConn2 -- Three-Phase V-I Measurement/LConn2
  Three-Phase Breaker1/RConn1 -- Three-Phase V-I Measurement/LConn1
  Three-Phase Breaker2/RConn2 -- Three-Phase Series RLC Branch8/LConn2
  Three-Phase Series RLC Branch8/LConn1 -- Three-Phase Breaker2/RConn1
  Three-Phase Breaker2/RConn3 -- Three-Phase Series RLC Branch8/LConn3
  Ground1/LConn1 -- Three-Phase Series RLC Branch8/RConn1 -- Three-Phase Series RLC Branch8/RConn2 -- Three-Phase Series RLC Branch8/RConn3
  Variant Subsystem3/RConn3 -- Three-Phase Series RLC Branch3/LConn3
  Variant Subsystem3/RConn2 -- Three-Phase Series RLC Branch3/LConn2
  Variant Subsystem3/RConn1 -- Three-Phase Series RLC Branch3/LConn1
  Variant Subsystem2/RConn2 -- Three-Phase Series RLC Branch2/LConn2
  Variant Subsystem2/RConn1 -- Three-Phase Series RLC Branch2/LConn1
  Variant Subsystem2/RConn3 -- Three-Phase Series RLC Branch2/LConn3
  Variant Subsystem1/RConn3 -- Three-Phase Series RLC Branch1/LConn3
  Variant Subsystem1/RConn2 -- Three-Phase Series RLC Branch1/LConn2
  Variant Subsystem1/RConn1 -- Three-Phase Series RLC Branch1/LConn1
  Three-Phase Series RLC Branch7/LConn1 -- Three-Phase V-I Measurement5/RConn1
  Three-Phase V-I Measurement5/RConn2 -- Three-Phase Series RLC Branch7/LConn2
  Three-Phase Series RLC Branch7/LConn3 -- Three-Phase V-I Measurement5/RConn3
  Controlled Voltage Source4/LConn1 -- Ground3/LConn1 -- Controlled Voltage Source5/LConn1 -- Controlled Voltage Source6/LConn1
  Three-Phase Breaker3/RConn3 -- Controlled Voltage Source5/RConn1
  Three-Phase Breaker3/RConn2 -- Controlled Voltage Source4/RConn1
  Three-Phase Breaker3/RConn1 -- Controlled Voltage Source6/RConn1
  Ground2/LConn1 -- Breaker1/RConn1
  Three-Phase Series RLC Branch5/RConn3 -- Three-Phase Series RLC Branch10/LConn3 -- Three-Phase Series RLC Branch9/LConn3
  Ground5/LConn1 -- Three-Phase Series RLC Branch10/RConn3 -- Three-Phase Series RLC Branch10/RConn2 -- Three-Phase Series RLC Branch10/RConn1 -- Three-Phase Series RLC Branch9/RConn3 -- Three-Phase Series RLC Branch9/RConn2 -- Three-Phase Series RLC Branch9/RConn1
  Three-Phase Series RLC Branch5/RConn2 -- Three-Phase Series RLC Branch9/LConn2 -- Three-Phase Series RLC Branch10/LConn2
  Three-Phase Series RLC Branch5/RConn1 -- Three-Phase Series RLC Branch9/LConn1 -- Three-Phase Series RLC Branch10/LConn1

== system mmc_model/dq_to_ab_g ==
  in : Inport
  wt : Inport  Port=2
  Demux1 : Demux  Outputs=2
  Demux16 : Demux  Outputs=2
  Mux11 : Mux
  Selector : Selector  InputPortWidth=4  IndexOptions=Index vector (dialog)  Indices=[1 3]  OutputSizes=1
  Selector1 : Selector  InputPortWidth=4  IndexOptions=Index vector (dialog)  Indices=[2 4]  OutputSizes=1
  Subsystem : Subsystem
  Subsystem1 : Subsystem
  out : Outport
  wires:
  Selector/1 -> Subsystem/1(dq)
  Demux16/2 -> Mux11/3
  in/1 -> Selector1/1, Selector/1
  Subsystem/1(alpha_beta) -> Demux16/1
  Demux16/1 -> Mux11/1
  Mux11/1 -> out/1
  wt/1 -> Subsystem1/2(wt), Subsystem/2(wt)
  Selector1/1 -> Subsystem1/1(dq)
  Subsystem1/1(alpha_beta) -> Demux1/1
  Demux1/1 -> Mux11/2
  Demux1/2 -> Mux11/4

== system mmc_model/dq_to_ab_m ==
  in : Inport
  wt : Inport  Port=2
  Demux1 : Demux  Outputs=2
  Demux16 : Demux  Outputs=2
  Mux11 : Mux
  Selector : Selector  InputPortWidth=4  IndexOptions=Index vector (dialog)  Indices=[1 2]  OutputSizes=1
  Selector1 : Selector  InputPortWidth=4  IndexOptions=Index vector (dialog)  Indices=[3 4]  OutputSizes=1
  Subsystem : Subsystem
  Subsystem1 : Subsystem
  out : Outport
  wires:
  Selector/1 -> Subsystem/1(dq)
  in/1 -> Selector1/1, Selector/1
  Subsystem/1(alpha_beta) -> Demux16/1
  Demux16/1 -> Mux11/1
  Mux11/1 -> out/1
  wt/1 -> Subsystem1/2(wt), Subsystem/2(wt)
  Selector1/1 -> Subsystem1/1(dq)
  Subsystem1/1(alpha_beta) -> Demux1/1
  Demux1/1 -> Mux11/3
  Demux1/2 -> Mux11/4
  Demux16/2 -> Mux11/2

== system mmc_model/dq_to_ab_ns ==
  in : Inport
  wt : Inport  Port=2
  Demux1 : Demux  Outputs=2
  Demux16 : Demux  Outputs=2
  Mux11 : Mux
  Selector : Selector  InputPortWidth=4  IndexOptions=Index vector (dialog)  Indices=[1 3]  OutputSizes=1
  Selector1 : Selector  InputPortWidth=4  IndexOptions=Index vector (dialog)  Indices=[2 4]  OutputSizes=1
  Subsystem : Subsystem
  Subsystem1 : Subsystem
  out : Outport
  wires:
  Selector/1 -> Subsystem/1(dq)
  Demux16/2 -> Mux11/3
  in/1 -> Selector1/1, Selector/1
  Subsystem/1(alpha_beta) -> Demux16/1
  Demux16/1 -> Mux11/1
  Mux11/1 -> out/1
  wt/1 -> Subsystem1/2(wt), Subsystem/2(wt)
  Selector1/1 -> Subsystem1/1(dq)
  Subsystem1/1(alpha_beta) -> Demux1/1
  Demux1/1 -> Mux11/2
  Demux1/2 -> Mux11/4

== system mmc_model/CPU/Current Limiting Control ==
  note: 1) Add Subsystem or Model blocks as valid variant choices.
      | 2) You cannot connect blocks at this level. At simulation, connectivity is automatically
      | determined, based on the active variant and port name matching.
  dm_ref : Inport
  i_ref : Inport  Port=2
  i : Inport  Port=3
  v_pcc : Inport  Port=4
  v_pcc_lp : Inport  Port=5
  w : Inport  Port=6
  enable : Inport  Port=7
  i0 : Inport  Port=8
  Adaptive VI : Subsystem  VariantControl=ctrl.machine.ictrl.sel==5
  Current Control : Subsystem  VariantControl=ctrl.machine.ictrl.sel==3
  Current Limiting Control : Subsystem  VariantControl=ctrl.machine.ictrl.sel==4
  Open Loop : Subsystem  VariantControl=ctrl.machine.ictrl.sel==0
  Safety Filter : Subsystem  VariantControl=ctrl.machine.ictrl.sel==1
  Safety Filter B only : Subsystem  VariantControl=ctrl.machine.ictrl.sel==2
  dm : Outport
  v_pcc_f : Outport  Port=2
  dm_corr : Outport  Port=3
  dv_corr : Outport  Port=4
  lambda : Outport  Port=5

== system mmc_model/CPU/GFM Control ==
  note: 1) Add Subsystem or Model blocks as valid variant choices.
      | 2) You cannot connect blocks at this level. At simulation, connectivity is automatically
      | determined, based on the active variant and port name matching.
  pq_ref : Inport
  pq : Inport  Port=2
  w : Inport  Port=3
  wt : Inport  Port=4
  v_pcc_lp : Inport  Port=5
  v_pcc_abs : Inport  Port=6
  antiwindup : Inport  Port=7
  enable : Inport  Port=8
  EDPC : Subsystem  VariantControl=ctrl.machine.gfm_sel == 0
  EDPC (modified) : Subsystem  VariantControl=ctrl.machine.gfm_sel == 2
  VSM : Subsystem  VariantControl=ctrl.machine.gfm_sel == 1
  m : Outport

== system mmc_model/CPU/PQ Calc ==
  v : Inport
  i : Inport  Port=2
  Gain2 : Gain  Gain=J  Multiplication=Matrix(K*u) (u vector)
  Mux : Mux  Inputs=2
  Product1 : Product  Multiplication=Matrix(*)
  Product2 : Product  Multiplication=Matrix(*)
  Transpose : Math  Operator=transpose
  Transpose1 : Math  Operator=transpose
  PQ : Outport
  wires:
  Gain2/1 -> Transpose1/1
  v/1 -> Transpose/1, Gain2/1
  i/1 -> Product2/2, Product1/2
  Product1/1 -> Mux/1
  Product2/1 -> Mux/2
  Transpose1/1 -> Product2/1
  Transpose/1 -> Product1/1
  Mux/1 -> PQ/1

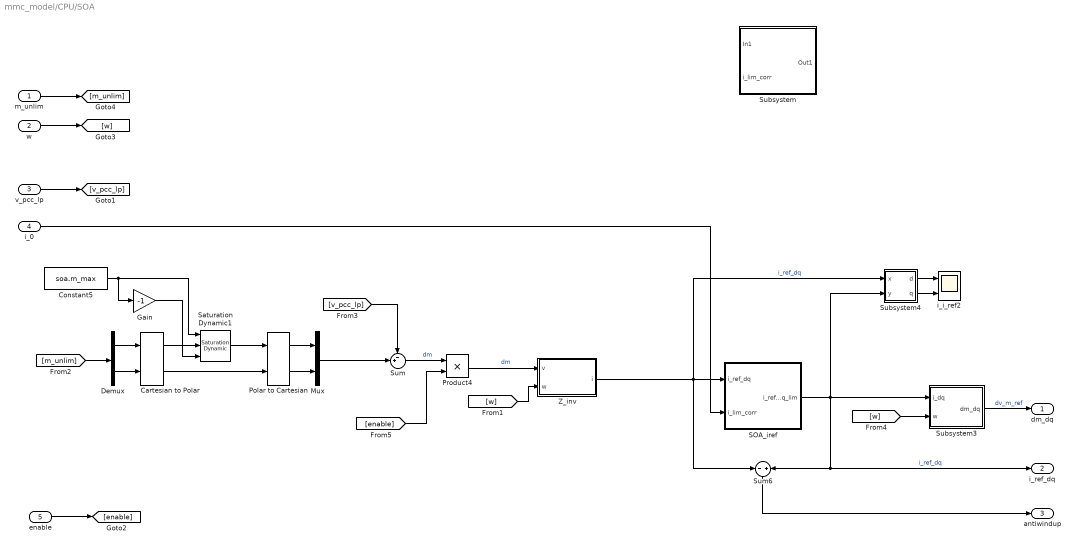
== system mmc_model/CPU/SOA ==
  m_unlim : Inport
  w : Inport  Port=2
  v_pcc_lp : Inport  Port=3
  i_0 : Inport  Port=4
  enable : Inport  Port=5
  Cartesian to Polar : simulink_extras/Transformations/Cartesian to Polar
  Constant5 : Constant  Value=soa.m_max
  Demux : Demux  Outputs=2
  Gain : Gain  Gain=-1
  Mux : Mux  Inputs=2
  Polar to Cartesian : simulink_extras/Transformations/Polar to Cartesian
  Product4 : Product
  SOA_iref : Subsystem
  Saturation Dynamic1 : simulink/Discontinuities/Saturation Dynamic  OutMin=[]  OutMax=[]  OutDataTypeStr=Inherit: Same as second input  OutDataType=fixdt(1, 16)  OutScaling=2^-10  DoSatur=off
  Subsystem : Subsystem
  Subsystem3 : Subsystem
  Subsystem4 : Subsystem
  Sum : Sum  Inputs=-+|
  Sum6 : Sum  Inputs=-|+
  Z_inv : Subsystem
  i_i_ref2 : Scope  NumInputPorts=2
  dm_dq : Outport
  i_ref_dq : Outport  Port=2
  antiwindup : Outport  Port=3
  wires:
  Z_inv/1(i) -> SOA_iref/1(i_ref_dq), Sum6/1, Subsystem4/1(x)  "i_ref_dq"
  SOA_iref/1(i_ref_dq_lim) -> i_ref_dq/1, Sum6/2, Subsystem3/1(i_dq), Subsystem4/2(y)  "i_ref_dq"
  Subsystem4/1(d) -> i_i_ref2/1
  Subsystem4/2(q) -> i_i_ref2/2
  w/1 -> [w]
  [w] -> Subsystem3/2(w)
  Subsystem3/1(dm_dq) -> dm_dq/1  "dv_m_ref"
  [w] -> Z_inv/2(w)
  m_unlim/1 -> [m_unlim]
  Sum6/1 -> antiwindup/1
  v_pcc_lp/1 -> [v_pcc_lp]
  Product4/1 -> Z_inv/1(v)  "dm"
  [v_pcc_lp] -> Sum/1
  i_0/1 -> SOA_iref/2(i_lim_corr)
  Cartesian to Polar/1 -> Saturation Dynamic1/2
  Constant5/1 -> Gain/1, Saturation Dynamic1/1
  Gain/1 -> Saturation Dynamic1/3
  Saturation Dynamic1/1 -> Polar to Cartesian/1
  Cartesian to Polar/2 -> Polar to Cartesian/2
  Polar to Cartesian/1 -> Mux/1
  Polar to Cartesian/2 -> Mux/2
  Mux/1 -> Sum/2
  Demux/2 -> Cartesian to Polar/2
  Demux/1 -> Cartesian to Polar/1
  [m_unlim] -> Demux/1
  enable/1 -> [enable]
  Sum/1 -> Product4/1  "dm"
  [enable] -> Product4/2

== system mmc_model/CPU/Subsystem ==
  x : Inport
  y : Inport  Port=2
  Demux : Demux  Outputs=2
  Demux1 : Demux  Outputs=2
  Mux1 : Mux  Inputs=2
  Mux2 : Mux  Inputs=2
  d : Outport
  q : Outport  Port=2
  wires:
  Mux2/1 -> q/1
  y/1 -> Demux1/1
  Demux/2 -> Mux2/1
  Demux1/2 -> Mux2/2
  Demux/1 -> Mux1/1
  Demux1/1 -> Mux1/2
  Mux1/1 -> d/1
  x/1 -> Demux/1

== system mmc_model/CPU/Subsystem1 ==
  x : Inport
  y : Inport  Port=2
  Demux : Demux  Outputs=2
  Demux1 : Demux  Outputs=2
  Mux1 : Mux  Inputs=2
  Mux2 : Mux  Inputs=2
  d : Outport
  q : Outport  Port=2
  wires:
  Mux2/1 -> q/1
  y/1 -> Demux1/1
  Demux/2 -> Mux2/1
  Demux1/2 -> Mux2/2
  Demux/1 -> Mux1/1
  Demux1/1 -> Mux1/2
  Mux1/1 -> d/1
  x/1 -> Demux/1

== system mmc_model/CPU/Subsystem2 ==
  x : Inport
  y : Inport  Port=2
  Demux : Demux  Outputs=2
  Demux1 : Demux  Outputs=2
  Mux1 : Mux  Inputs=2
  Mux2 : Mux  Inputs=2
  d : Outport
  q : Outport  Port=2
  wires:
  Mux2/1 -> q/1
  y/1 -> Demux1/1
  Demux/2 -> Mux2/1
  Demux1/2 -> Mux2/2
  Demux/1 -> Mux1/1
  Demux1/1 -> Mux1/2
  Mux1/1 -> d/1
  x/1 -> Demux/1

== system mmc_model/CPU/Subsystem3 ==
  x : Inport
  y : Inport  Port=2
  Demux : Demux  Outputs=2
  Demux1 : Demux  Outputs=2
  Mux1 : Mux  Inputs=2
  Mux2 : Mux  Inputs=2
  d : Outport
  q : Outport  Port=2
  wires:
  Mux2/1 -> q/1
  y/1 -> Demux1/1
  Demux/2 -> Mux2/1
  Demux1/2 -> Mux2/2
  Demux/1 -> Mux1/1
  Demux1/1 -> Mux1/2
  Mux1/1 -> d/1
  x/1 -> Demux/1

== system mmc_model/CPU/Subsystem5 ==
  x : Inport
  y : Inport  Port=2
  Demux : Demux  Outputs=2
  Demux1 : Demux  Outputs=2
  Mux1 : Mux  Inputs=2
  Mux2 : Mux  Inputs=2
  d : Outport
  q : Outport  Port=2
  wires:
  Mux2/1 -> q/1
  y/1 -> Demux1/1
  Demux/2 -> Mux2/1
  Demux1/2 -> Mux2/2
  Demux/1 -> Mux1/1
  Demux1/1 -> Mux1/2
  Mux1/1 -> d/1
  x/1 -> Demux/1

== system mmc_model/CPU/Subsystem6 ==
  x : Inport
  y : Inport  Port=2
  Demux : Demux  Outputs=2
  Demux1 : Demux  Outputs=2
  Mux1 : Mux  Inputs=2
  Mux2 : Mux  Inputs=2
  d : Outport
  q : Outport  Port=2
  wires:
  Mux2/1 -> q/1
  y/1 -> Demux1/1
  Demux/2 -> Mux2/1
  Demux1/2 -> Mux2/2
  Demux/1 -> Mux1/1
  Demux1/1 -> Mux1/2
  Mux1/1 -> d/1
  x/1 -> Demux/1

== system mmc_model/CPU/ab_to_ab0 ==
  v_pcc_f : Inport
  Constant8 : Constant  Value=0
  Demux : Demux  Outputs=2
  Mux7 : Mux  Inputs=3
  Out1 : Outport
  wires:
  Demux/1 -> Mux7/1
  Demux/2 -> Mux7/2
  Constant8/1 -> Mux7/3
  v_pcc_f/1 -> Demux/1
  Mux7/1 -> Out1/1

== system mmc_model/CPU/ab_to_ab1 ==
  v_pcc_f : Inport
  Constant8 : Constant  Value=0
  Demux : Demux  Outputs=2
  Mux7 : Mux  Inputs=3
  Out1 : Outport
  wires:
  Demux/1 -> Mux7/1
  Demux/2 -> Mux7/2
  Constant8/1 -> Mux7/3
  v_pcc_f/1 -> Demux/1
  Mux7/1 -> Out1/1

== system mmc_model/CPU/correction ==
  In1 : Inport
  Constant : Constant  Value=0.5
  Constant1 : Constant
  Delay : Delay  DelayLength=1  InitialCondition=0
  Product : Product
  Product1 : Product
  Sum1 : Sum  Inputs=|+-
  Sum2 : Sum  Inputs=++|
  Out1 : Outport
  wires:
  Delay/1 -> Product1/2
  Sum2/1 -> Product/1
  Sum1/1 -> Out1/1
  Product/1 -> Sum1/1
  Constant/1 -> Sum2/2, Product1/1
  In1/1 -> Delay/1, Product/2
  Product1/1 -> Sum1/2
  Constant1/1 -> Sum2/1

== system mmc_model/CPU/droop ==
  w : Inport
  u_abs : Inport  Port=2
  Constant11 : Constant  Value=pq_ctrl.vg_ref
  Constant13 : Constant  Value=pq_ctrl.f_ref
  Low-Pass Filter (Discrete or Continuous)1 : eeGeneralControl/Low-Pass Filter (Discrete or Continuous)  K=1  T=0.02  B=inf  A=-inf  init_option=Inherited from block input  x0=0  Ts=-1
  Low-Pass Filter (Discrete or Continuous)5 : eeGeneralControl/Low-Pass Filter (Discrete or Continuous)  K=1  T=0.02  B=inf  A=-inf  init_option=Inherited from block input  x0=0  Ts=-1
  Mux1 : Mux  Inputs=2
  Saturation : Saturate  UpperLimit=1  LowerLimit=-1
  Saturation1 : Saturate  UpperLimit=1  LowerLimit=-1
  Sum2 : Sum  Inputs=|+-
  Sum5 : Sum  Inputs=|+-
  fP Droop : Gain  Gain=-1/pq_ctrl.fp_droop
  uQ Droop : Gain  Gain=1/pq_ctrl.uq_droop
  PQ_ref : Outport
  wires:
  Constant11/1 -> Sum5/2
  fP Droop/1 -> Saturation/1
  Low-Pass Filter (Discrete or Continuous)1/1 -> Sum2/1
  Sum5/1 -> uQ Droop/1
  Mux1/1 -> PQ_ref/1  "PQ_ref"
  uQ Droop/1 -> Saturation1/1
  Low-Pass Filter (Discrete or Continuous)5/1 -> Sum5/1
  Sum2/1 -> fP Droop/1
  Constant13/1 -> Sum2/2
  u_abs/1 -> Low-Pass Filter (Discrete or Continuous)5/1
  w/1 -> Low-Pass Filter (Discrete or Continuous)1/1
  Saturation/1 -> Mux1/1
  Saturation1/1 -> Mux1/2

== system mmc_model/CPU/feedforward ==
  i_dq : Inport
  w : Inport  Port=2
  Gain : Gain  Gain=J  Multiplication=Matrix(K*u) (u vector)
  Gain1 : Gain  Gain=grid.tr.l
  Gain2 : Gain  Gain=grid.tr.r
  Product : Product
  Sum8 : Sum  Inputs=++|
  dm_dq : Outport
  wires:
  Gain1/1 -> Sum8/2
  Sum8/1 -> dm_dq/1  "dm_dq"
  Product/1 -> Gain/1
  Gain/1 -> Gain1/1  "dm_dq"
  w/1 -> Product/1
  i_dq/1 -> Gain2/1, Product/2
  Gain2/1 -> Sum8/1
